simulink model "MotoriRastgard"  (R2014a)
settings: Solver=ode45  StartTime=0.0  StopTime=2  RelTol=1e-3
libraries: powerlib x13, powerlib_meascontrol x1
settings Model: Creator=pc6229  LastModifiedBy=pc6229

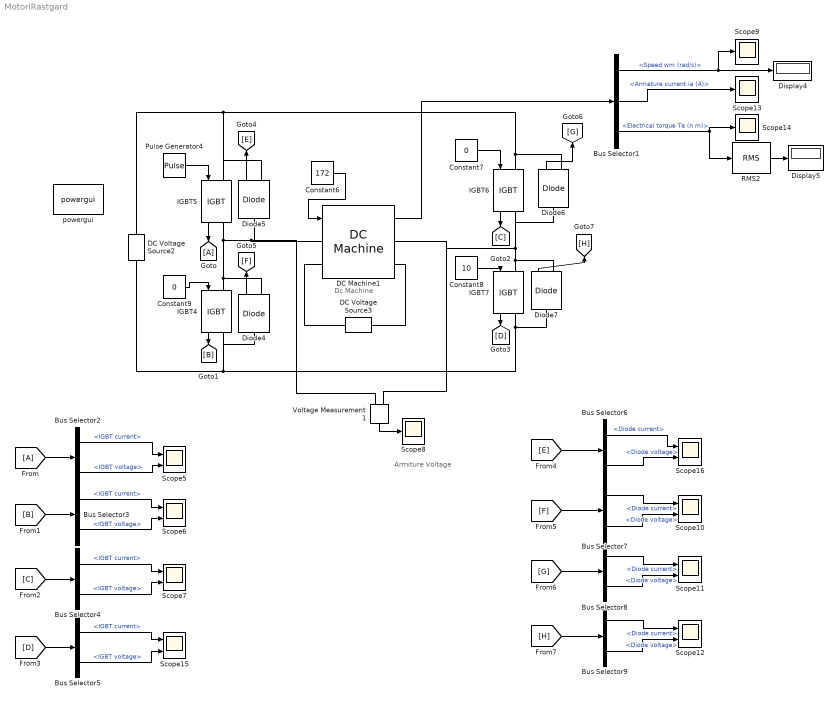
== system MotoriRastgard ==
  note: Armiture Voltage
  note: Dc Machine
  Bus Selector1 : BusSelector  OutputSignals=Speed wm (rad/s),Armature current ia (A),Electrical torque Te (n m)
  Bus Selector{2..5} (4 alike) : BusSelector  OutputSignals=IGBT current,IGBT voltage
  Bus Selector{6..9} (4 alike) : BusSelector  OutputSignals=Diode current,Diode voltage
  Constant6 : Constant  Value=172
  Constant7 : Constant  Value=0
  Constant8 : Constant  Value=10
  Constant9 : Constant  Value=0
  DC Machine1 : powerlib/Machines/DC Machine  PresetModel=No  MechanicalLoad=Torque TL  FieldType=Wound  ShowDetailedParameters=on  MeasurementBus=off  RLa="[ 0.4  0.028]"  RLf=[ 110 150]  Laf=1.8  MachineConstant=Torque constant (N.m/A)  Ke=1.8  Kt=1.8  J=1  Bm=0  Tf=0  w0=1  Ifinit=1  TsPowergui=0  TsBlock=-1
  DC Voltage Source2 : powerlib/Electrical Sources/DC Voltage Source  Amplitude=600  Measurements=None
  DC Voltage Source3 : powerlib/Electrical Sources/DC Voltage Source  Amplitude=162  Measurements=None
  Diode{4..7} (4 alike) : powerlib/Power Electronics/Diode  Ron=0.001  Lon=0  Vf=0.8  IC=0  UseSnubber=off  Rs=500  Cs=250e-9  Measurements=on
  Display4 : Display
  Display5 : Display
  IGBT{4..7} (4 alike) : powerlib/Power Electronics/IGBT  Ron=0.001  Lon=0  Vf=1  Tf=1e-6  Tt=2e-6  IC=0  Rs=1e5  Cs=inf  Measurements=on
  Pulse Generator4 : DiscretePulseGenerator  PulseType=Time based  Amplitude=10  Period=0.002  PulseWidth=60
  RMS2 : powerlib_meascontrol/Measurements/RMS  TrueRMS=on  Freq=60  RMSInit=120  Ts=0
  Scope{5..7,10..12,15..16} (8 alike) : Scope  NumInputPorts=2
      Scope10 settings: YMin=-50~-5  YMax=500~5  SaveName=ScopeData9
      Scope11 settings: YMin=-5~-5  YMax=5~5  SaveName=ScopeData10
      Scope12 settings: YMin=-5~-5  YMax=5~5  SaveName=ScopeData11
      Scope15 settings: YMin=-5~-5  YMax=5~5  SaveName=ScopeData7
      Scope16 settings: YMin=-5~-5  YMax=5~5  SaveName=ScopeData8
      Scope5 settings: YMin=-100~-5  YMax=500~5  SaveName=ScopeData12
      Scope6 settings: YMin=-5~-100  YMax=5~700  SaveName=ScopeData13
      Scope7 settings: YMin=-5~-5  YMax=5~5  SaveName=ScopeData14
  Scope{8..9,13..14} (4 alike) : Scope
      Scope13 settings: YMin=15  YMax=85  SaveName=ScopeData5
      Scope14 settings: SaveName=ScopeData6
      Scope8 settings: YMin=-100  YMax=700  SaveName=ScopeData15
      Scope9 settings: SaveName=ScopeData4
  Voltage Measurement1 : powerlib/Measurements/Voltage Measurement  PhasorSimulation=off  OutputType=Complex  PSBequivalent=0
  powergui : powerlib/powergui  Priority=1  SimulationMode=Discrete  SolverType=Tustin  SampleTime=50e-6  frequency=60  SPID=off  DisableSnubberDevices=off  DisableRonSwitches=off  DisableVfSwitches=off  SwTol=0  Interpol=off  DisplayEquations=off  Ts=0  methode=off  frequencyindice=0  Pbase=100e6  ErrMax=1e-4  Iterations=50  UnitsV=kV  UnitsW=MW  FunctionMessages=off  echomessages=off  HookPort=off  EnableUseOfTLC=off  x0status=blocks  RestoreLinks=warning  ResistiveCurrentMeasurement=off  Frange=[0:2:500]  Ylog=off  Xlog=on  ShowGrid=off  save=off  variable=ZData  structure=0  ZoomFFT=off  StartTime=0.0  cycles=1  DisplayStyle=1  fundamental=60  FreqAxis=off  MaxFrequency=1000  frequencyindicesteady=1  RmsSteady=1  display=off
  wires:
  Constant6/1 -> DC Machine1/1
  DC Machine1/1 -> Bus Selector1/1
  Bus Selector1/1 -> Scope9/1, Display4/1  "<Speed wm (rad/s)>"
  Bus Selector1/2 -> Scope13/1  "<Armature current ia (A)>"
  Constant7/1 -> IGBT6/1
  Constant8/1 -> IGBT7/1
  Bus Selector1/3 -> RMS2/1, Scope14/1  "<Electrical torque Te (n m)>"
  Constant9/1 -> IGBT4/1
  Pulse Generator4/1 -> IGBT5/1
  RMS2/1 -> Display5/1
  Voltage Measurement1/1 -> Scope8/1
  IGBT5/1 -> [A]
  IGBT4/1 -> [B]
  IGBT6/1 -> [C]
  IGBT7/1 -> [D]
  [A] -> Bus Selector2/1
  [B] -> Bus Selector3/1
  [C] -> Bus Selector4/1
  [D] -> Bus Selector5/1
  Bus Selector2/1 -> Scope5/1  "<IGBT current>"
  Bus Selector2/2 -> Scope5/2  "<IGBT voltage>"
  Bus Selector3/1 -> Scope6/1  "<IGBT current>"
  Bus Selector3/2 -> Scope6/2  "<IGBT voltage>"
  Bus Selector4/2 -> Scope7/2  "<IGBT voltage>"
  Bus Selector4/1 -> Scope7/1  "<IGBT current>"
  Bus Selector5/1 -> Scope15/1  "<IGBT current>"
  Bus Selector5/2 -> Scope15/2  "<IGBT voltage>"
  Diode5/1 -> [E]
  Diode4/1 -> [F]
  Diode7/1 -> [H]
  Diode6/1 -> [G]
  [E] -> Bus Selector6/1
  [F] -> Bus Selector7/1
  [G] -> Bus Selector8/1
  [H] -> Bus Selector9/1
  Bus Selector6/1 -> Scope16/1  "<Diode current>"
  Bus Selector6/2 -> Scope16/2  "<Diode voltage>"
  Bus Selector7/1 -> Scope10/1  "<Diode current>"
  Bus Selector7/2 -> Scope10/2  "<Diode voltage>"
  Bus Selector8/1 -> Scope11/1  "<Diode current>"
  Bus Selector8/2 -> Scope11/2  "<Diode voltage>"
  Bus Selector9/1 -> Scope12/1  "<Diode current>"
  Bus Selector9/2 -> Scope12/2  "<Diode voltage>"
  connections:
  IGBT6/LConn1 -- Diode6/RConn1 -- Diode5/RConn1 -- IGBT5/LConn1 -- DC Voltage Source2/RConn1
  IGBT7/RConn1 -- Diode7/LConn1 -- Diode4/LConn1 -- IGBT4/RConn1 -- DC Voltage Source2/LConn1
  IGBT5/RConn1 -- DC Machine1/LConn1 -- Voltage Measurement1/LConn1 -- Diode5/LConn1 -- Diode4/RConn1 -- IGBT4/LConn1
  IGBT7/LConn1 -- Diode7/RConn1 -- Diode6/LConn1 -- IGBT6/RConn1 -- DC Machine1/RConn1 -- Voltage Measurement1/LConn2
  DC Machine1/LConn2 -- DC Voltage Source3/RConn1
  DC Machine1/RConn2 -- DC Voltage Source3/LConn1
